simulink model "Quaternions_Method_merge_gio_giusto"  (R2021b)
settings: Solver=FixedStepAuto  StartTime=0.0  StopTime=Time  FixedStep=1  RelTol=1e-13  AbsTol=1e-8
values from neighbouring files (symbols this model uses):
  a = 8.6251e+06    (= 8625100)    [Main.m]
  c = 299792*10^3    (= 299792000)    [Main.m]
  e = 0.1195    [Main.m]
  G = 6.67259 * 1e-11    (= 6.67259e-11)    [Main.m]
  H_0 = sqrt((g_1_0)^2 + (g_1_1)^2 + (h_1_1)^2)    [Main.m]
  i = 0.3815    [Main.m]
  MB = [2000; 0.3; 1; 0.12].*1e-2    [Main.m]
  mr = 1.2 * 0.0001    (= 0.00012)    [Main.m]
  muP = G*Mt    (= 398527110340000)    [Main.m]
  omega_0 = [om_x, om_y, om_z]    [Main.m]
  p_acc = deg2rad(5)    [Main.m]
  RD = 0.1*ones(1,10)    [Main.m]
  RS_MB = 0.5    [Main.m]
  RS_SP = 0.1    [Main.m]
  SP = [2000; 0.3; 1; 0.12].*1e-2    [Main.m]
  theta0 = 0    [Main.m]
  w_E = (2*pi)/(24*3600)    (= 7.27220521664e-05)    [Main.m]
undefined symbols (not defined in the file or in its folder): A_BN_0, A_rw, A_rw_star, H, magnitude, rho_d_MB, rho_d_SP, rho_s_MB, rho_s_SP, sig_b, sig_n, T, t_sample
libraries: matrix_library x23, vrlib x9, simulink_extras x2, simulink x2
(part 2 of 8)

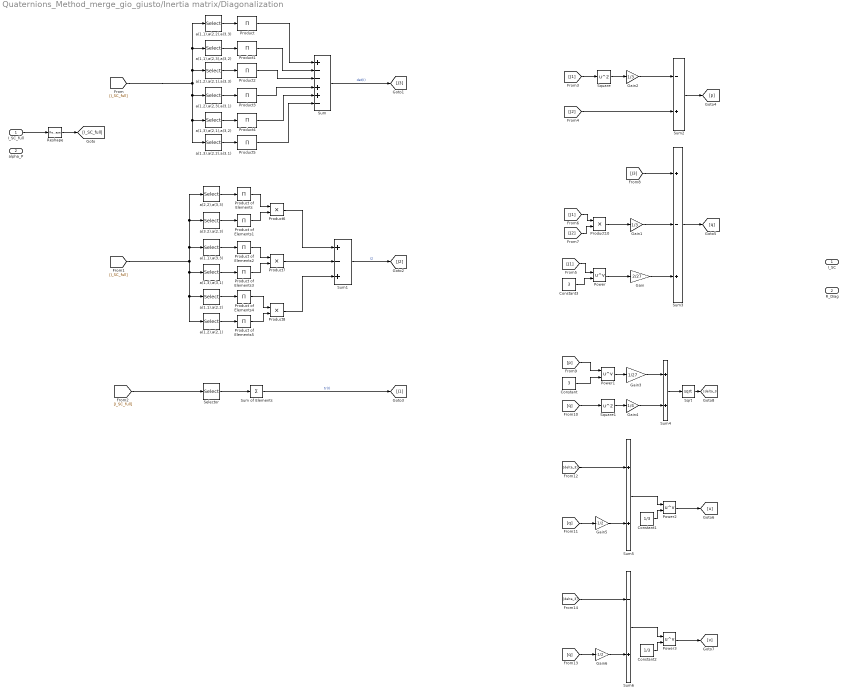
== system Quaternions_Method_merge_gio_giusto/Inertia matrix/Diagonalization ==
  I_SC_full : Inport
  alpha_P : Inport  Port=2
  Constant : Constant  Value=3
  Constant1 : Constant  Value=1/3
  Constant2 : Constant  Value=1/3
  Constant3 : Constant  Value=3
  Gain : Gain  Gain=2/27
  Gain1 : Gain  Gain=1/3
  Gain2 : Gain  Gain=1/3
  Gain3 : Gain  Gain=1/27
  Gain4 : Gain  Gain=1/4
  Gain5 : Gain  Gain=-1/2
  Gain6 : Gain  Gain=-1/2
  Power{,1..3} (4 alike) : Math  Operator=pow  SaturateOnIntegerOverflow=on
  Product{,1..5} (6 alike) : Product  Inputs=1  SaturateOnIntegerOverflow=on  OutDataTypeStr=Inherit: Same as first input
  Product of Elements{,1..5} (6 alike) : Product  Inputs=*
  Product{6..8,10} (4 alike) : Product
  Reshape : Reshape  OutputDimensionality=Column vector (2-D)
  Selector : Selector  InputPortWidth=9  IndexOptions=Index vector (dialog)  Indices=[1 5 9]  OutputSizes=1
  Sqrt : Sqrt  SaturateOnIntegerOverflow=on
  Square : Math  Operator=square  SaturateOnIntegerOverflow=on
  Square1 : Math  Operator=square  SaturateOnIntegerOverflow=on
  Sum : Sum  Inputs=+--++-  SaturateOnIntegerOverflow=on
  Sum of Elements : Sum  Inputs=+
  Sum1 : Sum  Inputs=+-+
  Sum2 : Sum  Inputs=-+
  Sum3 : Sum  Inputs=+-+
  Sum4 : Sum
  Sum5 : Sum
  Sum6 : Sum  Inputs=-+
  a(1,1),a(2,2) : Selector  InputPortWidth=9  IndexOptions=Index vector (dialog)  Indices=[1 3]  OutputSizes=1
  a(1,1),a(2,2),a(3,3) : Selector  InputPortWidth=9  IndexOptions=Index vector (dialog)  Indices=[1 5 9]  OutputSizes=1
  a(1,1),a(2,3),a(3,2) : Selector  InputPortWidth=9  IndexOptions=Index vector (dialog)  Indices=[1 6 8]  OutputSizes=1
  a(1,2),a(2,1) : Selector  InputPortWidth=9  IndexOptions=Index vector (dialog)  Indices=[1 3]  OutputSizes=1
  a(1,2),a(2,1),a(3,3) : Selector  InputPortWidth=9  IndexOptions=Index vector (dialog)  Indices=[2 4 9]  OutputSizes=1
  a(1,2),a(2,3),a(3,1) : Selector  InputPortWidth=9  IndexOptions=Index vector (dialog)  Indices=[3 4 8]  OutputSizes=1
  a(1,3),a(2,1),a(3,2) : Selector  InputPortWidth=9  IndexOptions=Index vector (dialog)  Indices=[2 6 7]  OutputSizes=1
  a(1,3),a(2,2),a(3,1) : Selector  InputPortWidth=9  IndexOptions=Index vector (dialog)  Indices=[3 5 7]  OutputSizes=1
  a(1,3),a(3,1) : Selector  InputPortWidth=9  IndexOptions=Index vector (dialog)  Indices=[1 3]  OutputSizes=1
  a(1.1),a(3,3) : Selector  InputPortWidth=9  IndexOptions=Index vector (dialog)  Indices=[1 3]  OutputSizes=1
  a(2,2),a(3,3) : Selector  InputPortWidth=9  IndexOptions=Index vector (dialog)  Indices=[5 9]  OutputSizes=1
  a(3.2),a(2,3) : Selector  InputPortWidth=9  IndexOptions=Index vector (dialog)  Indices=[6 8]  OutputSizes=1
  I_SC : Outport
  R_Diag : Outport  Port=2
  wires:
  [I_SC_full] -> a(1,3),a(2,2),a(3,1)/1, a(1,3),a(2,1),a(3,2)/1, a(1,2),a(2,3),a(3,1)/1, a(1,1),a(2,2),a(3,3)/1, a(1,1),a(2,3),a(3,2)/1, a(1,2),a(2,1),a(3,3)/1
  Product2/1 -> Sum/3
  Product3/1 -> Sum/4
  a(1,2),a(2,1),a(3,3)/1 -> Product2/1
  a(1,1),a(2,3),a(3,2)/1 -> Product1/1
  Product/1 -> Sum/1
  a(1,3),a(2,2),a(3,1)/1 -> Product5/1
  a(1,1),a(2,2),a(3,3)/1 -> Product/1
  a(1,3),a(2,1),a(3,2)/1 -> Product4/1
  Product4/1 -> Sum/5
  Product1/1 -> Sum/2
  Product5/1 -> Sum/6
  a(1,2),a(2,3),a(3,1)/1 -> Product3/1
  I_SC_full/1 -> Reshape/1
  Reshape/1 -> [I_SC_full]
  Sum/1 -> [J3]  "det(I)"
  Product6/1 -> Sum1/1
  Product7/1 -> Sum1/2
  Product8/1 -> Sum1/3
  Sum1/1 -> [J2]  "I2"
  [I_SC_full] -> a(1,3),a(3,1)/1, a(1,1),a(2,2)/1, a(1,2),a(2,1)/1, a(1.1),a(3,3)/1, a(3.2),a(2,3)/1, a(2,2),a(3,3)/1
  [I_SC_full] -> Selector/1
  Selector/1 -> Sum of Elements/1
  a(2,2),a(3,3)/1 -> Product of Elements/1
  a(3.2),a(2,3)/1 -> Product of Elements1/1
  a(1.1),a(3,3)/1 -> Product of Elements2/1
  a(1,3),a(3,1)/1 -> Product of Elements3/1
  a(1,1),a(2,2)/1 -> Product of Elements4/1
  a(1,2),a(2,1)/1 -> Product of Elements5/1
  Product of Elements5/1 -> Product8/2
  Product of Elements4/1 -> Product8/1
  Product of Elements3/1 -> Product7/2
  Product of Elements2/1 -> Product7/1
  Product of Elements1/1 -> Product6/2
  Product of Elements/1 -> Product6/1
  Sum of Elements/1 -> [J1]  "tr(I)"
  [J2] -> Sum2/2
  [J1] -> Square/1
  Square/1 -> Gain2/1
  Gain2/1 -> Sum2/1
  Sum2/1 -> [p]
  [J2] -> Product10/2
  [J1] -> Product10/1
  [J3] -> Sum3/1
  Constant3/1 -> Power/2
  [J1] -> Power/1
  Power/1 -> Gain/1
  Product10/1 -> Gain1/1
  Gain1/1 -> Sum3/2
  Gain/1 -> Sum3/3
  Sum3/1 -> [q]
  [q] -> Square1/1
  [p] -> Power1/1
  Constant/1 -> Power1/2
  Square1/1 -> Gain4/1
  Power1/1 -> Gain3/1
  Gain4/1 -> Sum4/2
  Gain3/1 -> Sum4/1
  Sum4/1 -> Sqrt/1
  [q] -> Gain5/1
  Gain5/1 -> Sum5/2
  Sum5/1 -> Power2/1
  Constant1/1 -> Power2/2
  Power2/1 -> [u]
  Sqrt/1 -> [delta_3]
  [delta_3] -> Sum5/1
  [delta_3] -> Sum6/1
  Constant2/1 -> Power3/2
  Sum6/1 -> Power3/1
  [q] -> Gain6/1
  Power3/1 -> [v]
  Gain6/1 -> Sum6/2

== system Quaternions_Method_merge_gio_giusto/Inertia matrix/Main body ==
  m_MB : Inport
  a_MB : Inport  Port=2
  b_MB : Inport  Port=3
  h_MB : Inport  Port=4
  Constant : Constant  Value=0
  Gain : Gain  Gain=1/12
  Gain1 : Gain  Gain=1/12
  Gain2 : Gain  Gain=1/12
  Product : Product
  Product1 : Product
  Product2 : Product
  Reshape : Reshape  OutputDimensionality=Customize  OutputDimensions=[3,3]
  Square : Math  Operator=square  SaturateOnIntegerOverflow=on
  Square1 : Math  Operator=square  SaturateOnIntegerOverflow=on
  Square2 : Math  Operator=square  SaturateOnIntegerOverflow=on
  Sum : Sum
  Sum1 : Sum
  Sum2 : Sum
  Vector Concatenate : Concatenate  NumInputs=9
  I_MB : Outport
  wires:
  Constant/1 -> Vector Concatenate/2, Vector Concatenate/3, Vector Concatenate/7, Vector Concatenate/8, Vector Concatenate/6, Vector Concatenate/4
  Square/1 -> Sum2/1, Sum1/1
  Square1/1 -> Sum2/2, Sum/1
  Square2/1 -> Sum/2, Sum1/2
  Product1/1 -> Gain1/1
  Gain/1 -> Vector Concatenate/1
  Product2/1 -> Gain2/1
  Sum1/1 -> Product1/2
  m_MB/1 -> Product/1, Product2/1, Product1/1
  Sum2/1 -> Product2/2
  a_MB/1 -> Square/1
  Vector Concatenate/1 -> Reshape/1
  Sum/1 -> Product/2
  b_MB/1 -> Square1/1
  Gain1/1 -> Vector Concatenate/5
  Product/1 -> Gain/1
  Gain2/1 -> Vector Concatenate/9
  Reshape/1 -> I_MB/1
  h_MB/1 -> Square2/1

== system Quaternions_Method_merge_gio_giusto/Inertia matrix/SP_Rotation from SP principal to MB principal ==
  gamma_SP : Inport
  I_SP : Inport  Port=2
  Constant : Constant
  Demux : Demux  Outputs=9
  Gain : Gain  Gain=-1
  Gain1 : Gain  Gain=2
  Gain2 : Gain  Gain=1/2
  Ground : Ground
  Product : Product
  Reciprocal : Product  Inputs=/
  Reshape : Reshape  OutputDimensionality=Customize  OutputDimensions=[3,3]
  Sin : Trigonometry  Operator=cos
  Sin1 : Trigonometry
  Sin2 : Trigonometry  Operator=atan
  Sum : Sum  Inputs=+-
  Sum1 : Sum
  Terminator{,1..5} (6 alike) : Terminator
  Vector Concatenate : Concatenate  NumInputs=9
  R_SP : Outport
  alpha_P : Outport  Port=2
  wires:
  Vector Concatenate/1 -> Reshape/1
  Reshape/1 -> R_SP/1
  Constant/1 -> Vector Concatenate/1
  Ground/1 -> Vector Concatenate/7, Vector Concatenate/4, Vector Concatenate/3, Vector Concatenate/2
  gamma_SP/1 -> Sum1/1
  Gain/1 -> Vector Concatenate/6
  Sin/1 -> Vector Concatenate/5, Vector Concatenate/9
  Sin1/1 -> Gain/1, Vector Concatenate/8
  I_SP/1 -> Demux/1
  Demux/1 -> Terminator/1
  Demux/2 -> Terminator1/1
  Demux/3 -> Terminator2/1
  Demux/4 -> Terminator3/1
  Demux/5 -> Sum/1  "I22"
  Demux/6 -> Gain1/1  "I31"
  Demux/7 -> Terminator4/1
  Demux/8 -> Terminator5/1
  Demux/9 -> Sum/2  "I33"
  Sum/1 -> Reciprocal/1
  Reciprocal/1 -> Product/1
  Gain1/1 -> Product/2
  Product/1 -> Sin2/1
  Sin2/1 -> Gain2/1
  Gain2/1 -> alpha_P/1, Sum1/2
  Sum1/1 -> Sin1/1, Sin/1

== system Quaternions_Method_merge_gio_giusto/Inertia matrix/Solar panel ==
  note: The inertia matrix for the solar panels is for two solar panels since they are the same and they are on opposite sides the distance vector between the centers of mass are one the opposite of the other and in the transport theorem the sign does not matter since I need only the norm and the d'*d that has + sign anyway
      | Still the mass and all characteristics are about one solar panel
  m_SP : Inport
  a_SP : Inport  Port=2
  b_SP : Inport  Port=3
  h_SP : Inport  Port=4
  Gain : Gain  Gain=1/12
  Gain1 : Gain  Gain=1/12
  Gain2 : Gain  Gain=1/12
  Gain3 : Gain  Gain=2
  Ground : Ground
  Product : Product
  Product1 : Product
  Product2 : Product
  Reshape : Reshape  OutputDimensionality=Customize  OutputDimensions=[3,3]
  Square : Math  Operator=square  SaturateOnIntegerOverflow=on
  Square1 : Math  Operator=square  SaturateOnIntegerOverflow=on
  Square2 : Math  Operator=square  SaturateOnIntegerOverflow=on
  Sum : Sum
  Sum1 : Sum
  Sum2 : Sum
  Vector Concatenate : Concatenate  NumInputs=9
  I_SP : Outport
  wires:
  Vector Concatenate/1 -> Reshape/1
  m_SP/1 -> Product/1, Product2/1, Product1/1
  Product/1 -> Gain/1
  Gain/1 -> Vector Concatenate/1
  Product1/1 -> Gain1/1
  Product2/1 -> Gain2/1
  Gain2/1 -> Vector Concatenate/9
  h_SP/1 -> Square/1
  a_SP/1 -> Square1/1
  b_SP/1 -> Square2/1
  Sum/1 -> Product/2
  Sum1/1 -> Product1/2
  Sum2/1 -> Product2/2
  Ground/1 -> Vector Concatenate/2, Vector Concatenate/3, Vector Concatenate/7, Vector Concatenate/8, Vector Concatenate/6, Vector Concatenate/4
  Gain1/1 -> Vector Concatenate/5
  Reshape/1 -> Gain3/1
  Gain3/1 -> I_SP/1
  Square1/1 -> Sum1/2, Sum2/1
  Square2/1 -> Sum/2, Sum2/2
  Square/1 -> Sum/1, Sum1/1

== system Quaternions_Method_merge_gio_giusto/Inertia matrix/Transport theorem ==
  I_SP : Inport
  r_SP : Inport  Port=2
  m_SP : Inport  Port=3
  Constant : Constant  Value=eye(3)
  Dot Product : DotProduct  InputSameDT=on  OutDataTypeStr=Inherit: Inherit via internal rule
  Gain : Gain  Gain=2
  Matrix Multiply : Product  Multiplication=Matrix(*)
  Matrix Multiply1 : Product
  Product : Product
  Sum : Sum  Inputs=+-
  Sum1 : Sum
  Transpose : Math  Operator=transpose  SaturateOnIntegerOverflow=on
  I_SP_B : Outport
  wires:
  r_SP/1 -> Transpose/1, Dot Product/2, Dot Product/1, Matrix Multiply/2
  Transpose/1 -> Matrix Multiply/1
  Constant/1 -> Matrix Multiply1/1
  Matrix Multiply1/1 -> Sum/1
  Matrix Multiply/1 -> Sum/2
  Sum/1 -> Product/2
  m_SP/1 -> Gain/1
  Product/1 -> Sum1/2
  I_SP/1 -> Sum1/1
  Sum1/1 -> I_SP_B/1
  Dot Product/1 -> Matrix Multiply1/2
  Gain/1 -> Product/1

== system Quaternions_Method_merge_gio_giusto/Inertia matrix/gamma_SP ==
  R_diag : Inport
  S_B : Inport  Port=2
  Cos : Trigonometry  Operator=acos
  Demux : Demux  Outputs=3
  Gain : Gain  Gain=-1
  Matrix Multiply1 : Product  Multiplication=Matrix(*)
  Terminator : Terminator
  Terminator1 : Terminator
  gamma_SP : Outport
  wires:
  R_diag/1 -> Matrix Multiply1/1
  S_B/1 -> Matrix Multiply1/2
  Matrix Multiply1/1 -> Demux/1  "S_p_SP"
  Demux/1 -> Terminator/1
  Demux/2 -> Terminator1/1
  Demux/3 -> Gain/1
  Gain/1 -> Cos/1
  Cos/1 -> gamma_SP/1

== system Quaternions_Method_merge_gio_giusto/Inertia matrix/r_SP ==
  b_SP : Inport
  a_MB : Inport  Port=2
  Constant : Constant  Value=[1 0 0]
  Gain : Gain  Gain=1/2
  Gain1 : Gain  Gain=1/2
  Gain2 : Gain  Gain=-1
  Product : Product
  Reshape : Reshape  OutputDimensionality=Column vector (2-D)
  Sum : Sum
  r_SP1 : Outport
  r_SP2 : Outport  Port=2
  wires:
  Constant/1 -> Reshape/1
  a_MB/1 -> Gain/1
  b_SP/1 -> Gain1/1
  Gain1/1 -> Sum/1
  Gain/1 -> Sum/2
  Reshape/1 -> Product/1
  Sum/1 -> Product/2
  Gain2/1 -> r_SP2/1
  Product/1 -> r_SP1/1, Gain2/1

== system Quaternions_Method_merge_gio_giusto/Kalman Observer/A^ ==
  A : Inport
  L : Inport  Port=2
  C : Inport  Port=3
  Add : Sum  Inputs=+-
  Matrix Multiply : Product  Multiplication=Matrix(*)
  A^ : Outport
  wires:
  L/1 -> Matrix Multiply/1
  Add/1 -> A^/1
  Matrix Multiply/1 -> Add/2
  C/1 -> Matrix Multiply/2
  A/1 -> Add/1

== system Quaternions_Method_merge_gio_giusto/Kalman Observer/B^ ==
  B : Inport
  L : Inport  Port=2
  D : Inport  Port=3
  Add : Sum  Inputs=+-
  Matrix Multiply : Product  Multiplication=Matrix(*)
  B^ : Outport
  wires:
  Add/1 -> B^/1
  B/1 -> Add/1
  L/1 -> Matrix Multiply/1
  D/1 -> Matrix Multiply/2
  Matrix Multiply/1 -> Add/2

== system Quaternions_Method_merge_gio_giusto/Kalman Observer/L ==
  P : Inport
  C : Inport  Port=2
  V : Inport  Port=3
  Matrix Multiply : Product  Inputs=3  Multiplication=Matrix(*)
  Reciprocal : Product  Inputs=/  Multiplication=Matrix(*)
  Transpose : Math  Operator=transpose  SaturateOnIntegerOverflow=on
  L : Outport
  wires:
  Matrix Multiply/1 -> L/1
  P/1 -> Matrix Multiply/1
  C/1 -> Transpose/1
  Transpose/1 -> Matrix Multiply/2
  V/1 -> Reciprocal/1
  Reciprocal/1 -> Matrix Multiply/3

== system Quaternions_Method_merge_gio_giusto/Kalman Observer/Riccati ==
  A : Inport
  C : Inport  Port=2
  F : Inport  Port=3
  W : Inport  Port=4
  V : Inport  Port=5
  P_0 : Inport  Port=6
  Add : Sum  Inputs=++++
  Gain : Gain  Gain=-1
  Integrator : Integrator  InitialConditionSource=external
  Matrix Multiply : Product  Multiplication=Matrix(*)
  Matrix Multiply1 : Product  Multiplication=Matrix(*)
  Matrix Multiply2 : Product  Inputs=3  Multiplication=Matrix(*)
  Matrix Multiply3 : Product  Inputs=5  Multiplication=Matrix(*)
  Reciprocal : Product  Inputs=/  Multiplication=Matrix(*)
  Transpose : Math  Operator=transpose  SaturateOnIntegerOverflow=on
  Transpose1 : Math  Operator=transpose  SaturateOnIntegerOverflow=on
  Transpose2 : Math  Operator=transpose  SaturateOnIntegerOverflow=on
  P : Outport
  wires:
  Integrator/1 -> P/1, [P]
  A/1 -> [A]
  F/1 -> [F]
  W/1 -> [W]
  V/1 -> [V]
  C/1 -> [C]
  [P] -> Matrix Multiply/2
  [A] -> Matrix Multiply/1
  [P] -> Matrix Multiply1/1
  [A] -> Transpose/1
  Transpose/1 -> Matrix Multiply1/2
  [F] -> Matrix Multiply2/1
  [W] -> Matrix Multiply2/2
  Transpose1/1 -> Matrix Multiply2/3
  [P] -> Gain/1
  Gain/1 -> Matrix Multiply3/1
  [C] -> Transpose2/1
  Transpose2/1 -> Matrix Multiply3/2
  [V] -> Reciprocal/1
  Reciprocal/1 -> Matrix Multiply3/3
  [C] -> Matrix Multiply3/4
  [P] -> Matrix Multiply3/5
  [F] -> Transpose1/1
  Matrix Multiply/1 -> Add/1
  Matrix Multiply3/1 -> Add/4
  Matrix Multiply1/1 -> Add/2
  Matrix Multiply2/1 -> Add/3
  Add/1 -> Integrator/1
  [P_0] -> Integrator/2
  P_0/1 -> [P_0]

== system Quaternions_Method_merge_gio_giusto/Kinematics1/Creazione Matrice A_BN ==
  q_normalizzato : Inport
  Reshape : Reshape  OutputDimensionality=Customize  OutputDimensions=[3,3]
  Vector Concatenate : Concatenate  NumInputs=3
  column 1 : Subsystem
  column 2 : Subsystem
  column 3 : Subsystem
  A_BN : Outport
  wires:
  Reshape/1 -> A_BN/1
  q_normalizzato/1 -> column 3/1(q_normalizzato), column 1/1(q_normalizzato), column 2/1(q_normalizzato)
  column 1/1(Column 1) -> Vector Concatenate/1
  column 2/1(Column 2) -> Vector Concatenate/2
  column 3/1(Column 3) -> Vector Concatenate/3
  Vector Concatenate/1 -> Reshape/1

== system Quaternions_Method_merge_gio_giusto/Kinematics1/Creazione quaternione ==
  ω_BN : Inport
  A_BN_des : Inport  Port=2
  DCM to quaternion : Subsystem
  Demux : Demux  Outputs=3
  Gain : Gain  Gain=0.5
  Initial condition A_BN : Constant  Value=A_BN_0
  Integrator : Integrator  InitialConditionSource=external  InitialCondition=[0; 0; 0; 1]
  Matrix Multiply : Product  Multiplication=Matrix(*)
  Normalisation : Subsystem
  Reshape : Reshape  OutputDimensionality=Column vector (2-D)
  Subsystem : Subsystem
  q_normalizzato : Outport
  wires:
  Subsystem/1(OMEGA1) -> Gain/1
  Matrix Multiply/1 -> Integrator/1  "dq/dt"
  Gain/1 -> Matrix Multiply/1
  ω_BN/1 -> Demux/1
  Demux/1 -> Subsystem/1(om_x)
  Demux/2 -> Subsystem/2(om_y)
  Demux/3 -> Subsystem/3(om_z)
  Integrator/1 -> Reshape/1  "q(t)"
  Reshape/1 -> Normalisation/1(In1)
  DCM to quaternion/1(q) -> Integrator/2
  Normalisation/1(Out1) -> Matrix Multiply/2, [q_norm]  "q(t)"
  [q_norm] -> q_normalizzato/1
  Initial condition A_BN/1 -> DCM to quaternion/1(DCM)

== system Quaternions_Method_merge_gio_giusto/Kinematics1/Orbit Propagation ==
  A_BN : Inport
  Constant : Constant  Value=muP
  Constant1 : Constant  Value=e^2
  Constant2 : Constant
  Constant3 : Constant  Value=3
  Constant4 : Constant
  Constant5 : Constant  Value=3/2
  Cos : Trigonometry  Operator=cos
  Divide : Product  Inputs=*/
  Divide1 : Product  Inputs=*/
  Divide2 : Product  Inputs=*/
  Gain : Gain  Gain=a
  Gain1 : Gain  Gain=e
  Integrator : Integrator  InitialCondition=theta0
  MatrixMultiply : Product  Multiplication=Matrix(*)
  Product : Product
  Product1 : Product
  Sqrt : Sqrt  SaturateOnIntegerOverflow=on
  Square : Math  Operator=pow  SaturateOnIntegerOverflow=on
  Square1 : Math  Operator=square  SaturateOnIntegerOverflow=on
  Square2 : Math  Operator=pow  SaturateOnIntegerOverflow=on
  Sum : Sum  Inputs=+-
  Sum1 : Sum
  Terminator : Terminator
  vector : Subsystem
  theta : Outport
  n : Outport  Port=2
  r_N : Outport  Port=3
  wires:
  Constant2/1 -> Sum/1
  Constant1/1 -> Sum/2
  Sum/1 -> Square2/1, Gain/1
  Gain/1 -> Divide/1
  Constant4/1 -> Sum1/1
  Sum1/1 -> Square1/1, Divide/2
  Gain1/1 -> Sum1/2
  Cos/1 -> Gain1/1
  Integrator/1 -> Cos/1, theta/1, vector/1(theta)  "theta"
  Divide1/1 -> Sqrt/1
  Constant/1 -> Divide1/1
  Square/1 -> Divide1/2
  Divide/1 -> Product1/1, Square/1  "R"
  Constant3/1 -> Square/2
  Sqrt/1 -> Product/1, n/1  "n"
  Square1/1 -> Product/2
  Constant5/1 -> Square2/2
  Product/1 -> Divide2/1
  Divide2/1 -> Integrator/1  "theta_dot"
  vector/1(Vector) -> Product1/2
  A_BN/1 -> MatrixMultiply/1
  Product1/1 -> r_N/1, MatrixMultiply/2  "rN"
  Square2/1 -> Divide2/2
  MatrixMultiply/1 -> Terminator/1  "rB"

== system Quaternions_Method_merge_gio_giusto/Kinematics1/Relative_Attitude ==
  A_BN : Inport
  theta : Inport  Port=2
  A_LN : Subsystem
  A_LN1 : Subsystem  Commented=on
  MatrixMultiply : Product  Multiplication=Matrix(*)
  Transpose : Math  Operator=transpose  SaturateOnIntegerOverflow=on
  A_BL : Outport
  A_L/N : Outport  Port=2
  wires:
  Transpose/1 -> MatrixMultiply/2
  MatrixMultiply/1 -> A_BL/1  "A_BL"
  A_LN/1(A_LN) -> Transpose/1, A_L/N/1
  A_BN/1 -> MatrixMultiply/1
  theta/1 -> A_LN/1(theta)

== system Quaternions_Method_merge_gio_giusto/Sensors/Gyroscopes ==
  note: gyro model: STIM300
  omega : Inport
  Integrator : Integrator
  Mux1 : Mux  Inputs=3
  Mux2 : Mux  Inputs=3
  Reshape : Reshape  OutputDimensionality=Column vector (2-D)
  Reshape1 : Reshape  OutputDimensionality=Column vector (2-D)
  Sum : Sum  Inputs=+++
  "b1 " : RandomNumber  Variance=sig_b  Seed=1  SampleTime=t_sample
  b2 : RandomNumber  Variance=sig_b  Seed=2  SampleTime=t_sample
  b3 : RandomNumber  Variance=sig_b  Seed=3  SampleTime=t_sample
  n1 : RandomNumber  Variance=sig_n  Seed=4  SampleTime=t_sample
  n2 : RandomNumber  Variance=sig_n  Seed=5  SampleTime=t_sample
  n3 : RandomNumber  Variance=sig_n  Seed=6  SampleTime=t_sample
  omega_m : Outport
  wires:
  Integrator/1 -> Sum/1
  "b1 "/1 -> Mux1/1
  b2/1 -> Mux1/2
  b3/1 -> Mux1/3
  n3/1 -> Mux2/3
  n2/1 -> Mux2/2
  n1/1 -> Mux2/1
  Mux1/1 -> Reshape/1
  Mux2/1 -> Reshape1/1
  Sum/1 -> omega_m/1
  omega/1 -> Sum/2
  Reshape/1 -> Integrator/1
  Reshape1/1 -> Sum/3

== system Quaternions_Method_merge_gio_giusto/Sensors/Magnetometer1 ==
  A_BN : Inport
  b_N : Inport  Port=2
  "Magnetometer " : Subsystem
  b_B computation : Subsystem
  model to reality difference : Subsystem
  b_B : Outport
  wires:
  "Magnetometer "/1(A_BN*_filtered) -> b_B computation/1(A_BN*), model to reality difference/2(A_BN*)
  A_BN/1 -> model to reality difference/1(A_BN), "Magnetometer "/1(A_BN)
  b_N/1 -> b_B computation/2(b_N), model to reality difference/3(b_N)
  b_B computation/1(b_B) -> b_B/1
  "Magnetometer "/2(A_BN*_not_filtered) -> model to reality difference/4(A_BN*1)

== system Quaternions_Method_merge_gio_giusto/Sensors/Sun sensor ==
  note: redwire space, digital sun sensor +/- 64°
  S_N : Inport
  A_BN : Inport  Port=2
  Add : Sum  Inputs=+-
  Add1 : Sum  Inputs=+-
  Constant : Constant  Value=0.25*pi/180
  Constant1 : Constant
  Constant2 : Constant  Value=0.25*pi/180
  Constant3 : Constant  Value=0.25*pi/180
  Delay1 : Delay  DelayLength=1
  Discrete Derivative : simulink/Discrete/Discrete Derivative  gainval=T^-1  ICPrevScaledInput=0.0  OutMin=[]  OutMax=[]  OutDataType=fixdt(1, 16)  OutScaling=2^-10  DoSatur=off
  Gain : Gain  Gain=-1
  Gain1 : Gain  Gain=-1
  Gain2 : Gain  Gain=-1
  Matrix Multiply : Product  Multiplication=Matrix(*)
  Matrix Multiply1 : Product  Multiplication=Matrix(*)
  Product : Product
  Product1 : Product
  Product2 : Product
  Random Number : RandomNumber  Variance=0.6*pi/180  SampleTime=t_sample
  Random Number1 : RandomNumber  Variance=0.6*pi/180  SampleTime=t_sample
  Random Number2 : RandomNumber  Variance=0.6*pi/180  SampleTime=t_sample
  Reshape : Reshape  OutputDimensionality=Customize  OutputDimensions=[3,3]
  Scope : Scope
  Vector Concatenate : Concatenate  NumInputs=9
  S_B : Outport
  wires:
  S_N/1 -> Matrix Multiply1/2
  Random Number/1 -> Product/2
  Constant/1 -> Product/1
  Matrix Multiply/1 -> Add1/1
  Discrete Derivative/1 -> Delay1/1
  Add1/1 -> Add/1, Discrete Derivative/1, S_B/1
  Constant1/1 -> Vector Concatenate/8, Vector Concatenate/5, Vector Concatenate/1
  Constant2/1 -> Product1/1
  Random Number1/1 -> Product1/2
  Random Number2/1 -> Product2/2
  Constant3/1 -> Product2/1
  Product2/1 -> Vector Concatenate/4, Gain/1
  Gain/1 -> Vector Concatenate/2
  Product1/1 -> Vector Concatenate/3, Gain2/1
  Gain1/1 -> Vector Concatenate/6
  Product/1 -> Gain1/1, Vector Concatenate/9
  Gain2/1 -> Vector Concatenate/7
  Delay1/1 -> Add1/2
  Reshape/1 -> Matrix Multiply/1
  Vector Concatenate/1 -> Reshape/1
  A_BN/1 -> Matrix Multiply1/1
  Matrix Multiply1/1 -> Add/2, Matrix Multiply/2
  Add/1 -> Scope/1

== system Quaternions_Method_merge_gio_giusto/Slew Manouevre "quaternion"/A_BN to quaternion ==
  " A_BN_Desiderd" : Inport
  Constant : Constant
  Demux1 : Demux  Outputs=9
  Divide : Product  Inputs=*/
  Divide1 : Product  Inputs=*/
  Divide2 : Product  Inputs=*/
  Gain : Gain  Gain=0.5
  Gain1 : Gain  Gain=4
  Gain2 : Gain  Gain=4
  Gain3 : Gain  Gain=4
  Mux : Mux
  Reshape : Reshape  OutputDimensionality=Column vector (2-D)
  Reshape1 : Reshape  OutputDimensionality=Column vector (2-D)
  Square Root : Sqrt  SaturateOnIntegerOverflow=on
  Sum : Sum  Inputs=|+|+|+|+|
  Sum1 : Sum  Inputs=|+|-|
  Sum2 : Sum  Inputs=|+|-|
  Sum3 : Sum  Inputs=|+|-|
  q_desiderd : Outport
  wires:
  [A33] -> Sum/4
  Mux/1 -> Reshape/1
  [q4] -> Gain3/1
  Gain1/1 -> Divide/2
  Divide/1 -> Mux/1
  [q4] -> Gain2/1
  [A13] -> Sum2/2
  Gain3/1 -> Divide2/2
  Reshape/1 -> q_desiderd/1
  Gain/1 -> Mux/4, [q4]
  Demux1/4 -> [A12]
  [A12] -> Sum3/1
  Divide2/1 -> Mux/3
  Sum3/1 -> Divide2/1
  Gain2/1 -> Divide1/2
  Sum2/1 -> Divide1/1
  [A31] -> Sum2/1
  Sum1/1 -> Divide/1
  Divide1/1 -> Mux/2
  [q4] -> Gain1/1
  Square Root/1 -> Gain/1
  Constant/1 -> Sum/1
  Sum/1 -> Square Root/1
  [A32] -> Sum1/2
  Demux1/2 -> [A21]
  Demux1/6 -> [A32]
  [A22] -> Sum/3
  [A23] -> Sum1/1
  " A_BN_Desiderd"/1 -> Reshape1/1
  Demux1/1 -> [A11]
  [A11] -> Sum/2
  Reshape1/1 -> Demux1/1
  [A21] -> Sum3/2
  Demux1/8 -> [A23]
  Demux1/5 -> [A22]
  Demux1/9 -> [A33]
  Demux1/3 -> [A31]
  Demux1/7 -> [A13]

== system Quaternions_Method_merge_gio_giusto/Slew Manouevre "quaternion"/Creation of Q_euler1 ==
  q_desired : Inport
  Demux : Demux
  Gain{,1..3,5..6} (6 alike) : Gain  Gain=-1
  Mux{,1..3} (4 alike) : Mux
  Reshape : Reshape  OutputDimensionality=Column vector (2-D)
  Reshape{1..3,5} (4 alike) : Reshape  OutputDimensionality=Row vector (2-D)
  Reshape4 : Reshape  OutputDimensionality=Customize  OutputDimensions=[4,4]
  Vector Concatenate : Concatenate  NumInputs=4
  Q_desired : Outport
  wires:
  Reshape4/1 -> Q_desired/1
  Vector Concatenate/1 -> Reshape4/1
  Reshape3/1 -> Vector Concatenate/3
  Reshape2/1 -> Vector Concatenate/2
  Reshape1/1 -> Vector Concatenate/1
  Gain6/1 -> Mux2/2
  [q1] -> Gain6/1
  [q4] -> Mux1/2
  Gain2/1 -> Mux1/1
  [q3] -> Gain2/1
  Gain5/1 -> Mux2/4
  Mux2/1 -> Reshape3/1
  [q3] -> Gain5/1
  [q2] -> Mux2/1
  [q4] -> Mux2/3
  Gain3/1 -> Mux1/4
  Mux1/1 -> Reshape2/1
  [q2] -> Gain3/1
  [q1] -> Mux1/3
  Mux/1 -> Reshape1/1
  Gain/1 -> Mux/3
  [q3] -> Mux/2
  [q4] -> Mux/1
  Gain1/1 -> Mux/4
  [q1] -> Gain1/1
  [q2] -> Gain/1
  Demux/4 -> [q4]
  Demux/3 -> [q3]
  Demux/2 -> [q2]
  Demux/1 -> [q1]
  Reshape/1 -> Demux/1
  q_desired/1 -> Reshape/1
  Reshape5/1 -> Vector Concatenate/4
  [q1] -> Mux3/1
  Mux3/1 -> Reshape5/1
  [q2] -> Mux3/2
  [q4] -> Mux3/4
  [q3] -> Mux3/3

== system Quaternions_Method_merge_gio_giusto/State/q to g ==
  q : Inport
  Demux : Demux
  Mux : Mux  Inputs=3
  Product : Product
  Product1 : Product
  Product2 : Product
  Reciprocal : Product  Inputs=/
  Reshape : Reshape  OutputDimensionality=Column vector (2-D)
  g : Outport
  wires:
  q/1 -> Demux/1
  Demux/1 -> [q1]
  Demux/2 -> [q2]
  Demux/3 -> [q3]
  Demux/4 -> [q4]
  [q4] -> Reciprocal/1
  Mux/1 -> Reshape/1
  Reshape/1 -> g/1
  [q1] -> Product/2
  Reciprocal/1 -> Product/1, Product1/1, Product2/1
  Product/1 -> Mux/1
  Product1/1 -> Mux/2
  [q2] -> Product1/2
  [q3] -> Product2/2
  Product2/1 -> Mux/3

== system Quaternions_Method_merge_gio_giusto/Sun Pointing 1/Pointing error with DCM ==
  A_B_N from attitude determination : Inport
  S_N : Inport  Port=2
  A_B_N from Euler : Inport  Port=3
  Add : Sum  Inputs=+|-
  Desired attitude : Subsystem
  Detected pointing error : Subsystem
  Real pointing error : Subsystem
  Difference between real and detected pointing error : Outport
  real error DCM : Outport  Port=2
  Detected error DCM : Outport  Port=3
  wires:
  A_B_N from attitude determination/1 -> Detected pointing error/2(A_B_N from attitude determination)
  Add/1 -> Difference between real and detected pointing error/1
  A_B_N from Euler/1 -> Real pointing error/1(" A_B_N from Euler")
  Desired attitude/1(Desired A_B_N) -> Real pointing error/2(Desired A_B_N), Detected pointing error/1(Desired A_B_N)
  Detected pointing error/1(detected pointing error) -> Detected error DCM/1, Add/2
  Real pointing error/1(real pointing error) -> real error DCM/1, Add/1
  S_N/1 -> Desired attitude/1(S_N)

== system Quaternions_Method_merge_gio_giusto/Sun Pointing 1/Pointing error with quaternions ==
  A_B_N from attitude determination : Inport
  S_N : Inport  Port=2
  A_B_N from Euler : Inport  Port=3
  A_B_N from Euler to quaternion : Subsystem
  A_B_N from attitude det to quaternion2 : Subsystem
  Add : Sum  Inputs=+|-
  Add1 : Sum  Inputs=+|-
  Desired attitude : Subsystem
  Desired attitude to quaternion1 : Subsystem
  real pointing error : Outport
  detected pointing error : Outport  Port=2
  q_euler : Outport  Port=3
  q_desired : Outport  Port=4
  A_BN_des : Outport  Port=5
  wires:
  S_N/1 -> Desired attitude/1(S_N)
  A_B_N from attitude determination/1 -> A_B_N from attitude det to quaternion2/1(DCM)
  A_B_N from Euler/1 -> A_B_N from Euler to quaternion/1(A_B_N from Euler)
  Desired attitude/1(Desired A_B_N) -> [A_BN_des], Desired attitude to quaternion1/1(DCM)
  A_B_N from Euler to quaternion/1(q_euler) -> q_euler/1, Add/1
  Desired attitude to quaternion1/1(q) -> q_desired/1, Add1/1, Add/2
  A_B_N from attitude det to quaternion2/1(q) -> Add1/2
  Add/1 -> real pointing error/1
  Add1/1 -> detected pointing error/1
  [A_BN_des] -> A_BN_des/1

== system Quaternions_Method_merge_gio_giusto/Attitude determination/q to DCM/q_cross ==
  q_vect : Inport
  Demux : Demux  Outputs=3
  Gain : Gain  Gain=-1
  Gain1 : Gain  Gain=-1
  Gain2 : Gain  Gain=-1
  Ground : Ground
  Reshape : Reshape  OutputDimensionality=Customize  OutputDimensions=[3,3]
  Vector Concatenate : Concatenate  NumInputs=9
  q_cross : Outport
  wires:
  q_vect/1 -> Demux/1
  Reshape/1 -> q_cross/1
  Vector Concatenate/1 -> Reshape/1
  Ground/1 -> Vector Concatenate/1, Vector Concatenate/5, Vector Concatenate/9
  Gain/1 -> Vector Concatenate/3
  Gain1/1 -> Vector Concatenate/4
  Gain2/1 -> Vector Concatenate/8
  Demux/1 -> [q1]
  Demux/2 -> [q2]
  Demux/3 -> [q3]
  [q3] -> Vector Concatenate/2
  [q2] -> Gain/1
  [q3] -> Gain1/1
  [q1] -> Vector Concatenate/6
  [q2] -> Vector Concatenate/7
  [q1] -> Gain2/1

== system Quaternions_Method_merge_gio_giusto/Enviroment/Magnetic torque /Creation of parasitic torque ==
  Constant : Constant  Value=0.01
  Constant1 : Constant  Value=0.05
  Constant2 : Constant  Value=0.01
  Mux : Mux  Inputs=3
  Reshape : Reshape  OutputDimensionality=Column vector (2-D)
  m : Outport
  wires:
  Constant/1 -> Mux/1
  Constant1/1 -> Mux/2
  Constant2/1 -> Mux/3
  Mux/1 -> Reshape/1
  Reshape/1 -> m/1

== system Quaternions_Method_merge_gio_giusto/Enviroment/Magnetic torque /Magnetic field in body frame ==
  A_B_N : Inport
  R : Inport  Port=2
  r_LVLH : Inport  Port=3
  Add : Sum  Commented=on  Inputs=+++
  Add1 : Sum  Commented=on  Inputs=+|-
  Clock : Clock
  Constant : Constant  Commented=on  Value=3
  Constant1 : Constant  Commented=on  Value=H_0
  Constant2 : Constant  Commented=on  Value=3
  Constant3 : Constant  Value=G
  Constant4 : Constant  Value=H
  Demux : Demux  Commented=on  Outputs=3
  Direction of M field : Subsystem  Commented=on
  Divide : Product  Commented=on  Inputs=*/
  Dot Product : DotProduct  Commented=on  InputSameDT=on  OutDataTypeStr=Inherit: Inherit via internal rule
  Gain : Gain  Commented=on  Gain=3
  Goto1 : Goto  Commented=on  GotoTag=R
  MATLAB Function : MATLAB Function  TreatAsAtomicUnit=on
  Math Function : Math  Commented=on  Operator=pow  SaturateOnIntegerOverflow=on
  Math Function1 : Math  Commented=on  Operator=magnitude^2  SaturateOnIntegerOverflow=on
  Math Function2 : Math  Commented=on  Operator=magnitude^2  SaturateOnIntegerOverflow=on
  Math Function3 : Math  Commented=on  Operator=magnitude^2  SaturateOnIntegerOverflow=on
  Math Function4 : Math  Commented=on  Operator=pow  SaturateOnIntegerOverflow=on
  MatrixMultiply : Product  Multiplication=Matrix(*)
  Normalize Vector : vrlib/Utilities/Normalize Vector  Commented=on  maxzero=0
  Product : Product  Commented=on
  Product1 : Product  Commented=on
  Product2 : Product  Commented=on
  Reshape : Reshape  Commented=on  OutputDimensionality=Column vector (2-D)
  Reshape1 : Reshape  OutputDimensionality=Column vector (2-D)
  Scope : Scope
  Sqrt : Sqrt  Commented=on  SaturateOnIntegerOverflow=on
  b_B : Outport
  b_N : Outport  Port=2
  wires:
  Normalize Vector/1 -> Product1/1, Dot Product/1
  Demux/2 -> Math Function2/1
  Constant1/1 -> Product/2
  Constant/1 -> Math Function4/2
  Demux/1 -> Math Function1/1
  MatrixMultiply/1 -> b_B/1
  Math Function1/1 -> Add/1
  Demux/3 -> Math Function3/1
  Divide/1 -> Product2/1
  Add/1 -> Sqrt/1
  Math Function/1 -> Divide/2
  Product1/1 -> Gain/1
  Math Function3/1 -> Add/3
  Product/1 -> Divide/1
  Direction of M field/1(m_vect) -> Add1/2, Dot Product/2
  Math Function4/1 -> Product/1
  Add1/1 -> Product2/2
  Math Function2/1 -> Add/2
  Gain/1 -> Add1/1
  Dot Product/1 -> Product1/2
  Sqrt/1 -> Math Function/1
  Reshape/1 -> Demux/1
  Constant2/1 -> Math Function/2
  A_B_N/1 -> [A_BN]
  [A_BN] -> MatrixMultiply/1
  r_LVLH/1 -> MATLAB Function/1(r_LVLH)
  R/1 -> MATLAB Function/2(r)
  Clock/1 -> MATLAB Function/3(t)
  MATLAB Function/1(b_N) -> Reshape1/1
  Constant3/1 -> MATLAB Function/4(G)
  Constant4/1 -> MATLAB Function/5(H)
  Reshape1/1 -> Scope/1, b_N/1, MatrixMultiply/2

== system Quaternions_Method_merge_gio_giusto/Enviroment/Solar Radiation Perturbation/Areas ==
  MB : Inport
  Demux : Demux
  Mux : Mux  Inputs=3
  Product1 : Product
  Product2 : Product
  Product4 : Product
  Terminator : Terminator
  A_vect : Outport
  wires:
  Product2/1 -> Mux/2  "a*h"
  Product4/1 -> Mux/1  "b*h"
  MB/1 -> Demux/1
  Product1/1 -> Mux/3  "a*b"
  Demux/1 -> Terminator/1
  Demux/2 -> [a]
  Demux/3 -> [b]
  Demux/4 -> [h]
  [b] -> Product4/1
  [h] -> Product4/2
  [h] -> Product2/2
  [b] -> Product1/2
  [a] -> Product2/1
  [a] -> Product1/1
  Mux/1 -> A_vect/1

== system Quaternions_Method_merge_gio_giusto/Enviroment/Solar Radiation Perturbation/Force ==
  note: y, -y, y, -y
  note: x,y,z, -x,-y.-z
  SB : Inport
  MB : Inport  Port=2
  SP : Inport  Port=3
  Constant1 : Constant  Value=1358
  Constant2 : Constant  Value=RD
  Constant3 : Constant  Value=c
  Constant6 : Constant  Value=1358
  Constant7 : Constant  Value=c
  MB Forces : Subsystem
  N_MB : Constant  Value=[1 0 0;0 1 0;0 0 1;-1 0 0; 0 -1 0; 0 0 -1]
  Product1 : Product
  Product8 : Product
  Reciprocal : Product  Inputs=/
  Reciprocal1 : Product  Inputs=/
  Reshape4 : Reshape  OutputDimensionality=Column vector (2-D)
  Reshape5 : Reshape  OutputDimensionality=Column vector (2-D)
  SB1 : InportShadow
  SP Forces : Subsystem
  Selector : Selector  InputPortWidth=10  IndexOptions=Index vector (dialog)  Indices=[1 2 3 4 5 6]  OutputSizes=1
  Selector21 : Selector  InputPortWidth=10  IndexOptions=Index vector (dialog)  Indices=[7 8 9 10]  OutputSizes=1
  Transpose : Math  Operator=transpose  SaturateOnIntegerOverflow=on
  Transpose1 : Math  Operator=transpose  SaturateOnIntegerOverflow=on
  normali SP : Constant  Value=[0 1 0; 0 -1 0; 0 1 0; 0 -1 0]
  F_MB : Outport
  F_SP : Outport  Port=2
  A_MB : Outport  Port=3
  prodsca_MB : Outport  Port=4
  prodscal_SP1 : Outport  Port=5
  wires:
  Reshape5/1 -> [RD_SP]
  SB/1 -> Transpose/1
  Reshape4/1 -> MB Forces/3(RD_MB)
  Constant6/1 -> Product8/1
  Product8/1 -> MB Forces/1(P)
  Transpose/1 -> MB Forces/2(S_B)
  Reciprocal/1 -> Product8/2
  Constant7/1 -> Reciprocal/1
  MB/1 -> MB Forces/5(M_B)
  Selector/1 -> Reshape4/1
  Selector21/1 -> Reshape5/1
  Constant2/1 -> Selector21/1, Selector/1
  N_MB/1 -> MB Forces/4(N_MB)
  MB Forces/1(F_MB) -> F_MB/1
  MB Forces/2(A_MB) -> A_MB/1
  MB Forces/3(prodsca_MB) -> prodsca_MB/1
  SP Forces/1(F_SP) -> F_SP/1
  SP Forces/2(prodscal_SP1) -> prodscal_SP1/1
  Product1/1 -> SP Forces/1(P)
  Reciprocal1/1 -> Product1/2
  Constant1/1 -> Product1/1
  Constant3/1 -> Reciprocal1/1
  [RD_SP] -> SP Forces/3(RD_SP)
  normali SP/1 -> SP Forces/4(N_SP)
  SP/1 -> SP Forces/5(SP)
  Transpose1/1 -> SP Forces/2(S_B)
  SB1/1 -> Transpose1/1

== system Quaternions_Method_merge_gio_giusto/Enviroment/Solar Radiation Perturbation/Force MB ==
  P : Inport
  NMB_true : Inport  Port=2
  A_vect : Inport  Port=3
  rho_d_MB : Inport  Port=4
  rho_s_MB : Inport  Port=5
  S_B : Inport  Port=6
  Add : Sum  Inputs=-+
  Add1 : Sum
  Add2 : Sum
  Constant : Constant
  Constant{1..4} (4 alike) : Constant  Value=[1 1 1]
  Gain : Gain  Gain=-1
  Gain1 : Gain  Gain=2
  Gain2 : Gain  Gain=2/3
  Matrix Multiply{,1..3} (4 alike) : Product  Multiplication=Matrix(*)
  Product : Product  Inputs=4
  Product1 : Product
  Product2 : Product
  Product3 : Product
  Reshape{,1..3} (4 alike) : Reshape  OutputDimensionality=Row vector (2-D)
  Reshape4 : Reshape  OutputDimensionality=Column vector (2-D)
  Subsystem : Subsystem
  F_MB : Outport
  wires:
  Product/1 -> F_MB/1
  P/1 -> [P]
  NMB_true/1 -> [NMB_true]
  A_vect/1 -> [A_vect]
  rho_d_MB/1 -> [rho_d_MB]
  rho_s_MB/1 -> [rho_s_MB]
  S_B/1 -> [S_B]
  [P] -> Gain/1
  Gain/1 -> Product/1
  [NMB_true] -> Subsystem/2(N_MB)
  [S_B] -> Subsystem/1(S_B)
  Subsystem/1(Out1) -> [dot_NMB_SB]
  [rho_s_MB] -> Add/2
  Constant/1 -> Add/1
  Add/1 -> Product1/1
  [S_B] -> Product1/2
  [rho_s_MB] -> Gain1/1
  [dot_NMB_SB] -> Product2/2
  Gain1/1 -> Product2/1
  Product2/1 -> Add2/1
  Gain2/1 -> Add2/2
  [rho_d_MB] -> Gain2/1
  [NMB_true] -> Product3/2
  Product3/1 -> Add1/2
  Add1/1 -> Product/4
  Constant1/1 -> Reshape/1
  Matrix Multiply/1 -> Product3/1
  Add2/1 -> Matrix Multiply/1
  Reshape/1 -> Matrix Multiply/2
  Matrix Multiply1/1 -> Add1/1
  Product1/1 -> Matrix Multiply1/1
  Constant2/1 -> Reshape1/1
  Reshape1/1 -> Matrix Multiply1/2
  Reshape2/1 -> Matrix Multiply2/2
  Constant3/1 -> Reshape2/1
  Reshape3/1 -> Matrix Multiply3/2
  Constant4/1 -> Reshape3/1
  [A_vect] -> Reshape4/1
  Reshape4/1 -> Matrix Multiply2/1
  [dot_NMB_SB] -> Matrix Multiply3/1
  Matrix Multiply3/1 -> Product/3
  Matrix Multiply2/1 -> Product/2

== system Quaternions_Method_merge_gio_giusto/Enviroment/Solar Radiation Perturbation/Pressure ==
  Constant6 : Constant  Value=1358
  Constant7 : Constant  Value=c
  Product8 : Product
  Reciprocal : Product  Inputs=/
  P : Outport
  wires:
  Constant6/1 -> Product8/1
  Reciprocal/1 -> Product8/2
  Product8/1 -> P/1
  Constant7/1 -> Reciprocal/1

== system Quaternions_Method_merge_gio_giusto/Enviroment/Solar Radiation Perturbation/S_B dot N_MB ==
  N_MB : Inport
  S_B : Inport  Port=2
  Constant3 : Constant  Value=[1, 1, 1]
  Demux : Demux  Outputs=6
  If : If
  If Action Subsystem : Subsystem  TreatAsAtomicUnit=on
  If Action Subsystem1 : Subsystem  TreatAsAtomicUnit=on
  If Action Subsystem2 : Subsystem  TreatAsAtomicUnit=on
  If Action Subsystem3 : Subsystem  TreatAsAtomicUnit=on
  If Action Subsystem4 : Subsystem  TreatAsAtomicUnit=on
  If Action Subsystem5 : Subsystem  TreatAsAtomicUnit=on
  If1 : If
  If2 : If
  Matrix Multiply5 : Product  Multiplication=Matrix(*)
  Merge{,1..5} (6 alike) : Merge
  Mux : Mux  Inputs=3
  Product10 : Product
  Reshape{,1..4,12} (6 alike) : Reshape  OutputDimensionality=Column vector (2-D)
  Reshape11 : Reshape  OutputDimensionality=Row vector (2-D)
  Reshape5 : Reshape  OutputDimensionality=Customize  OutputDimensions=[3,3]
  Sum of Elements : Sum  Inputs=+  CollapseMode=Specified dimension  CollapseDim=2
  Terminator1 : Terminator
  Terminator2 : Terminator
  Terminator3 : Terminator
  Vector Concatenate : Concatenate  NumInputs=3
  MB_illuminated : Outport
  pointer : Outport  Port=2
  wires:
  Reshape12/1 -> Matrix Multiply5/2
  Matrix Multiply5/1 -> Product10/1
  Product10/1 -> Sum of Elements/1
  Reshape11/1 -> Matrix Multiply5/1
  Constant3/1 -> Reshape11/1
  S_B/1 -> Reshape12/1
  Sum of Elements/1 -> Reshape/1
  Reshape/1 -> Demux/1
  Demux/1 -> If/1
  If/1 -> If Action Subsystem/Action
  If/2 -> If Action Subsystem3/Action
  N_MB/1 -> [N_MB]
  [N_MB] -> Product10/2
  [N_MB] -> If Action Subsystem/1(NMB)
  Demux/4 -> Terminator1/1
  Demux/5 -> Terminator2/1
  Demux/6 -> Terminator3/1
  Demux/2 -> If1/1
  If1/1 -> If Action Subsystem1/Action
  [N_MB] -> If Action Subsystem3/1(NMB)
  [N_MB] -> If Action Subsystem1/1(NMB)
  If1/2 -> If Action Subsystem4/Action
  [N_MB] -> If Action Subsystem4/1(NMB)
  If Action Subsystem3/1(-x) -> Merge/2
  If Action Subsystem/1(x) -> Merge/1
  If Action Subsystem1/1(y) -> Merge1/1
  If Action Subsystem2/1(z) -> Merge2/1
  If Action Subsystem5/1(-z) -> Merge2/2
  Demux/3 -> If2/1
  If2/1 -> If Action Subsystem2/Action
  If2/2 -> If Action Subsystem5/Action
  [N_MB] -> If Action Subsystem2/1(NMB)
  [N_MB] -> If Action Subsystem5/1(NMB)
  Merge/1 -> Reshape1/1
  Merge1/1 -> Reshape2/1
  Merge2/1 -> Reshape3/1
  Reshape1/1 -> Vector Concatenate/1
  Reshape2/1 -> Vector Concatenate/2
  Reshape3/1 -> Vector Concatenate/3
  Vector Concatenate/1 -> Reshape5/1
  If Action Subsystem4/1(-y) -> Merge1/2
  If Action Subsystem/2(pointer) -> Merge4/1
  If Action Subsystem3/2(pointer) -> Merge4/2
  If Action Subsystem1/2(pointer) -> Merge5/1
  If Action Subsystem4/2(pointer) -> Merge5/2
  If Action Subsystem2/2(pointer) -> Merge3/1
  If Action Subsystem5/2(pointer) -> Merge3/2
  Merge4/1 -> Mux/1
  Merge5/1 -> Mux/2
  Merge3/1 -> Mux/3
  Mux/1 -> Reshape4/1
  Reshape4/1 -> pointer/1
  Reshape5/1 -> MB_illuminated/1

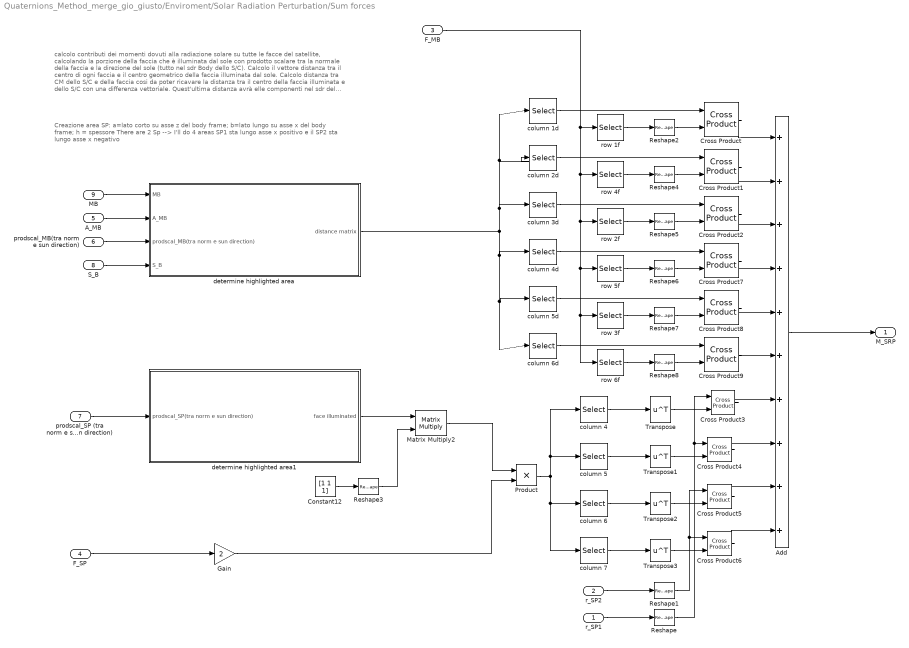
== system Quaternions_Method_merge_gio_giusto/Enviroment/Solar Radiation Perturbation/Sum forces ==
  note: Creazione area SP: a=lato corto su asse z del body frame; b=lato lungo su asse x del body frame; h = spessore
      | There are 2 Sp --> I'll do 4 areas
      | SP1 sta lungo asse x positivo e il SP2 sta lungo asse x negativo
  note: calcolo contributi dei momenti dovuti alla radiazione solare su tutte le facce del satellite, calcolando la porzione della faccia che è illuminata dal sole con prodotto scalare tra la normale della faccia e la direzione del sole (tutto nel sdr Body dello S/C). Calcolo il vettore distanza tra il centro di ogni faccia e il centro geometrico della faccia illuminata dal sole. Calcolo distanza tra CM dello S/C e della faccia cosi da poter ricavare la distanza tra il centro della faccia illuminata e dello S/C con una differenza vettoriale. Quest'ultima distanza avrà elle componenti nel sdr del S/C (body)
  r_SP1 : Inport
  r_SP2 : Inport  Port=2
  F_MB : Inport  Port=3
  F_SP : Inport  Port=4
  A_MB : Inport  Port=5
  prodscal_MB(tra norm e sun direction) : Inport  Port=6
  prodscal_SP (tra norm e sun direction) : Inport  Port=7
  S_B : Inport  Port=8
  MB : Inport  Port=9
  Add : Sum  Inputs=+|+|+|+|+|+|+|+|+|+
  Constant12 : Constant  Value=[1 1 1]
  Cross Product{,1..9} (10 alike) : matrix_library/Cross Product
      settings: SourceProductBaseCode=SL
  Gain : Gain  Gain=2
  Matrix Multiply2 : Product  Multiplication=Matrix(*)
  Product : Product
  Reshape{,1..2,4..8} (8 alike) : Reshape  OutputDimensionality=Column vector (2-D)
  Reshape3 : Reshape  OutputDimensionality=Row vector (2-D)
  Transpose{,1..3} (4 alike) : Math  Operator=transpose  SaturateOnIntegerOverflow=on
  column 1d : Selector  NumberOfDimensions=2  InputPortWidth=3  IndexOptions=Index vector (dialog),Index vector (dialog)  Indices=[1 2 3],1  OutputSizes=1,1
  column 2d : Selector  NumberOfDimensions=2  InputPortWidth=3  IndexOptions=Index vector (dialog),Index vector (dialog)  Indices=[1 2 3],2  OutputSizes=1,1
  column 3d : Selector  NumberOfDimensions=2  InputPortWidth=3  IndexOptions=Index vector (dialog),Index vector (dialog)  Indices=[1 2 3],3  OutputSizes=1,1
  column 4 : Selector  NumberOfDimensions=2  InputPortWidth=3  IndexOptions=Index vector (dialog),Index vector (dialog)  Indices=1,[1 2 3]  OutputSizes=1,1
  column 4d : Selector  NumberOfDimensions=2  InputPortWidth=3  IndexOptions=Index vector (dialog),Index vector (dialog)  Indices=[1 2 3],1  OutputSizes=1,1
  column 5 : Selector  NumberOfDimensions=2  InputPortWidth=3  IndexOptions=Index vector (dialog),Index vector (dialog)  Indices=2,[1 2 3]  OutputSizes=1,1
  column 5d : Selector  NumberOfDimensions=2  InputPortWidth=3  IndexOptions=Index vector (dialog),Index vector (dialog)  Indices=[1 2 3],2  OutputSizes=1,1
  column 6 : Selector  NumberOfDimensions=2  InputPortWidth=3  IndexOptions=Index vector (dialog),Index vector (dialog)  Indices=3,[1 2 3]  OutputSizes=1,1
  column 6d : Selector  NumberOfDimensions=2  InputPortWidth=3  IndexOptions=Index vector (dialog),Index vector (dialog)  Indices=[1 2 3],3  OutputSizes=1,1
  column 7 : Selector  NumberOfDimensions=2  InputPortWidth=3  IndexOptions=Index vector (dialog),Index vector (dialog)  Indices=4,[1 2 3]  OutputSizes=1,1
  determine highlighted area : Subsystem
  determine highlighted area1 : Subsystem
  row 1f : Selector  NumberOfDimensions=2  InputPortWidth=3  IndexOptions=Index vector (dialog),Index vector (dialog)  Indices=1,[1 2 3]  OutputSizes=1,1
  row 2f : Selector  NumberOfDimensions=2  InputPortWidth=3  IndexOptions=Index vector (dialog),Index vector (dialog)  Indices=2,[1 2 3]  OutputSizes=1,1
  row 3f : Selector  NumberOfDimensions=2  InputPortWidth=3  IndexOptions=Index vector (dialog),Index vector (dialog)  Indices=3,[1 2 3]  OutputSizes=1,1
  row 4f : Selector  NumberOfDimensions=2  InputPortWidth=3  IndexOptions=Index vector (dialog),Index vector (dialog)  Indices=4,[1 2 3]  OutputSizes=1,1
  row 5f : Selector  NumberOfDimensions=2  InputPortWidth=3  IndexOptions=Index vector (dialog),Index vector (dialog)  Indices=5,[1 2 3]  OutputSizes=1,1
  row 6f : Selector  NumberOfDimensions=2  InputPortWidth=3  IndexOptions=Index vector (dialog),Index vector (dialog)  Indices=6,[1 2 3]  OutputSizes=1,1
  M_SRP : Outport
  wires:
  prodscal_MB(tra norm e sun direction)/1 -> determine highlighted area/3(prodscal_MB(tra norm e sun direction))
  Add/1 -> M_SRP/1
  A_MB/1 -> determine highlighted area/2(A_MB)
  column 2d/1 -> Cross Product1/1
  column 1d/1 -> Cross Product/1
  column 3d/1 -> Cross Product2/1
  Cross Product1/1 -> Add/2
  Cross Product/1 -> Add/1
  Cross Product2/1 -> Add/3
  prodscal_SP (tra norm e sun direction)/1 -> determine highlighted area1/1(prodscal_SP(tra norm e sun direction))
  F_SP/1 -> Gain/1
  Gain/1 -> Product/2
  Reshape3/1 -> Matrix Multiply2/2
  Constant12/1 -> Reshape3/1
  determine highlighted area1/1(face illuminated) -> Matrix Multiply2/1
  Matrix Multiply2/1 -> Product/1
  r_SP1/1 -> Reshape/1
  r_SP2/1 -> Reshape1/1
  Product/1 -> column 7/1, column 6/1, column 4/1, column 5/1
  Cross Product3/1 -> Add/7
  Cross Product4/1 -> Add/8
  Cross Product5/1 -> Add/9
  Cross Product6/1 -> Add/10
  column 4/1 -> Transpose/1
  column 5/1 -> Transpose1/1
  column 6/1 -> Transpose2/1
  column 7/1 -> Transpose3/1
  Reshape/1 -> Cross Product3/1, Cross Product4/1
  Reshape1/1 -> Cross Product5/1, Cross Product6/1
  Transpose/1 -> Cross Product3/2
  Transpose1/1 -> Cross Product4/2
  Transpose2/1 -> Cross Product5/2
  Transpose3/1 -> Cross Product6/2
  Cross Product9/1 -> Add/6
  Cross Product7/1 -> Add/4
  Cross Product8/1 -> Add/5
  column 6d/1 -> Cross Product9/1
  column 4d/1 -> Cross Product7/1
  column 5d/1 -> Cross Product8/1
  determine highlighted area/1(distance matrix) -> column 2d/1, column 1d/1, column 3d/1, column 6d/1, column 5d/1, column 4d/1
  row 1f/1 -> Reshape2/1
  row 4f/1 -> Reshape4/1
  row 2f/1 -> Reshape5/1
  row 5f/1 -> Reshape6/1
  row 3f/1 -> Reshape7/1
  row 6f/1 -> Reshape8/1
  F_MB/1 -> row 6f/1, row 3f/1, row 5f/1, row 2f/1, row 4f/1, row 1f/1
  Reshape2/1 -> Cross Product/2
  Reshape4/1 -> Cross Product1/2
  Reshape5/1 -> Cross Product2/2
  Reshape6/1 -> Cross Product7/2
  Reshape7/1 -> Cross Product8/2
  Reshape8/1 -> Cross Product9/2
  MB/1 -> determine highlighted area/1(MB)
  S_B/1 -> determine highlighted area/4(S_B)

== system Quaternions_Method_merge_gio_giusto/Enviroment/Solar Radiation Perturbation/Sun position body ==
  A_B_N : Inport
  Clock : Clock
  Constant : Constant  Value=2*pi
  Constant1 : Constant  Value=365*24*60*60
  Constant2 : Constant  Value=23.45
  Degrees to Radians : simulink_extras/Transformations/Degrees to Radians
  MatrixMultiply : Product  Multiplication=Matrix(*)
  Mux : Mux  Inputs=3
  Product{,1..3} (4 alike) : Product
  Reciprocal : Product  Inputs=1
  Reshape : Reshape  OutputDimensionality=Column vector (2-D)
  Sin : Trigonometry  Operator=cos
  Sin1 : Trigonometry
  Sin2 : Trigonometry  Operator=cos
  Sin3 : Trigonometry
  S_B : Outport
  S_N : Outport  Port=2
  wires:
  Product3/1 -> Mux/3
  Degrees to Radians/1 -> Sin3/1, Sin2/1
  Constant1/1 -> Reciprocal/1
  Sin2/1 -> Product2/2
  Product/1 -> Product1/1  "n"
  Constant2/1 -> Degrees to Radians/1
  Product1/1 -> Sin/1, Sin1/1  "n*t"
  Product2/1 -> Mux/2
  Sin3/1 -> Product3/2
  Clock/1 -> Product1/2
  Sin1/1 -> Product3/1, Product2/1
  Constant/1 -> Product/1
  Sin/1 -> Mux/1
  Reciprocal/1 -> Product/2
  Mux/1 -> Reshape/1
  A_B_N/1 -> MatrixMultiply/1
  MatrixMultiply/1 -> S_B/1
  Reshape/1 -> S_N/1, MatrixMultiply/2
